simulink model "cartpendulum_compute_nom_traj"  (R2019b)
settings: Solver=VariableStepAuto  StartTime=0.0  StopTime=10.0  RelTol=1e-3
InitFcn:
  | init
values from neighbouring files (symbols this model uses):
  state0 = zeros(2,1)    [init.m]
  state0_1 = zeros(2,1)    [init.m]
settings Model: Creator=emanuele  LastModifiedBy=emanuele

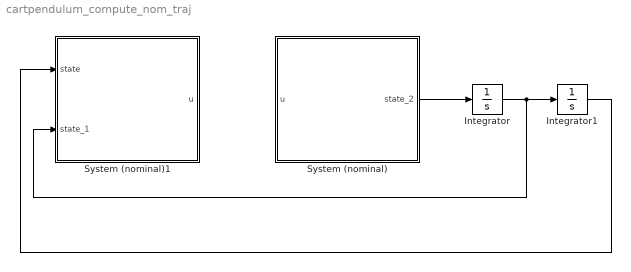
== system cartpendulum_compute_nom_traj ==
  Integrator : Integrator  InitialCondition=state0_1
  Integrator1 : Integrator  InitialCondition=state0
  System (nominal) : MATLAB Function  TreatAsAtomicUnit=on
  System (nominal)1 : MATLAB Function  TreatAsAtomicUnit=on
  wires:
  System (nominal)/1(state_2) -> Integrator/1
  Integrator/1 -> System (nominal)1/2(state_1), Integrator1/1
  Integrator1/1 -> System (nominal)1/1(state)

== matlab function cartpendulum_compute_nom_traj/System (nominal)1 ==
  data: state input; u output; state_1 input
function u = fcn(state,state_1)

u=0;

== matlab function cartpendulum_compute_nom_traj/System (nominal) ==
  data: state_2 output; u input
function state_2 = fcn(u)

state_2=[0;0];
